simulink model "gamma_controlled_ABS"  (Simulink 7.1)
settings: Solver=ode45  SolverMode=SingleTasking  StartTime=0.0  StopTime=5  RelTol=1e-3  AbsTol=1e-6
values from neighbouring files (symbols this model uses):
  Cs = 1050.0    (= 1050)    [rho_driven_suspension.m]
  Ks = 19960.0    (= 19960)    [rho_driven_suspension.m]
  Kw = 175500.0    (= 175500)    [rho_driven_suspension.m]
  ms = 427.0    (= 427)    [rho_driven_suspension.m]
  mw = 40.0    (= 40)    [rho_driven_suspension.m]
undefined symbols (not defined in the file or in its folder): Ct
settings Model: Creator=theShunainai  LastModifiedBy=theShunainai
settings DataIOCC: LimitDataPoints=off
settings OptimizationCC: BlockReduction=off  BooleanDataType=off
settings DebuggingCC: SaveWithParameterizedLinksMsg=none  SignalResolutionControl=TryResolveAllWithWarning  SolverPrmCheckMsg=none  MultiTaskDSMMsg=warning  MultiTaskCondExecSysMsg=none  StrictBusMsg=None
settings HardwareCC: TargetUnknown=on
settings RTWCC: IncludeERTFirstTime=on

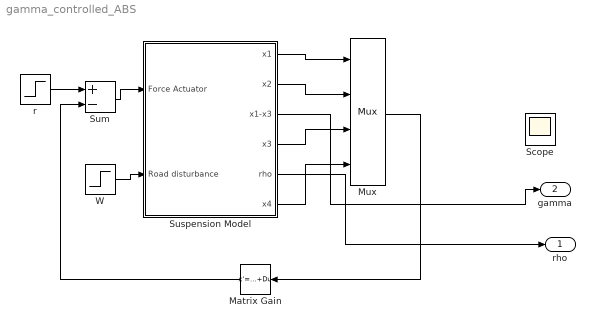
== system gamma_controlled_ABS ==
  Matrix Gain : StateSpace  Orientation=left  A=[]  B=[]  C=[]  D=K  mask(Matrix Gain){@1=-Kgamma}
      mask prompts: @1 "Gain matrix:"
      mask help: Matrix Gain.
      mask init:
      | K=@1;
      mask Help: Multiplies input vector by entered matrix to produce output vector (y=Au).
      mask Display: disp('K')
  Mux : Mux
  Scope : Scope
  Sum : Sum  Inputs=+-  SaturateOnIntegerOverflow=on  InputSameDT=on  OutDataTypeStr=Inherit: Same as first input
  Suspension Model : Subsystem
  W : Step  Time=0  After=-.1
  r : Step  Time=0  After=0
  rho : Outport  OutDataType=sfix(16)  OutScaling=2^0
  gamma : Outport  Port=2  OutDataType=sfix(16)  OutScaling=2^0
  wires:
  W/1 -> Suspension Model/2(Road disturbance)
  Sum/1 -> Suspension Model/1(Force Actuator)
  r/1 -> Sum/1
  Matrix Gain/1 -> Sum/2
  Mux/1 -> Matrix Gain/1
  Suspension Model/1(x1) -> Mux/1
  Suspension Model/2(x2) -> Mux/2
  Suspension Model/4(x3) -> Mux/3
  Suspension Model/6(x4) -> Mux/4
  Suspension Model/3(x1-x3) -> gamma/1
  Suspension Model/5(rho) -> rho/1

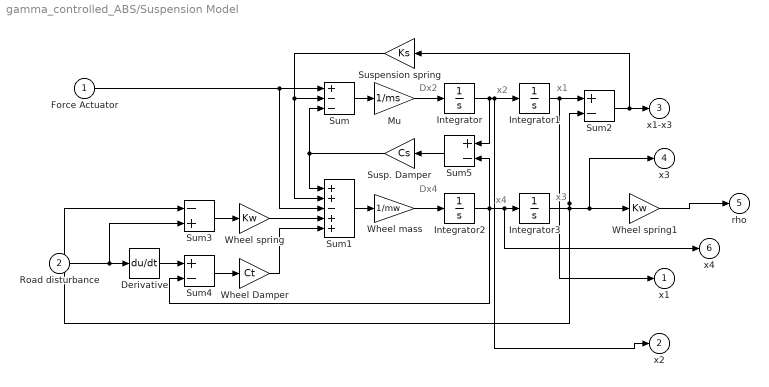
== system gamma_controlled_ABS/Suspension Model ==
  note: x3
  note: x4
  note: Dx4
  note: x1
  note: x2
  note: Dx2
  Force Actuator : Inport
  Road disturbance : Inport  Port=2
  Derivative : Derivative
  Integrator{,1..3} (4 alike) : Integrator
  Mu : Gain  Gain=1/ms  SaturateOnIntegerOverflow=on  OutDataTypeStr=Inherit: Same as input  ParamDataTypeStr=Inherit: Same as input
  Sum : Sum  Inputs=+--  SaturateOnIntegerOverflow=on  InputSameDT=on  OutDataTypeStr=Inherit: Same as first input
  Sum1 : Sum  Inputs=++-++  SaturateOnIntegerOverflow=on  InputSameDT=on  OutDataTypeStr=Inherit: Same as first input
  Sum2 : Sum  Inputs=+-  SaturateOnIntegerOverflow=on  InputSameDT=on  OutDataTypeStr=Inherit: Same as first input
  Sum3 : Sum  Inputs=-+  SaturateOnIntegerOverflow=on  InputSameDT=on  OutDataTypeStr=Inherit: Same as first input
  Sum4 : Sum  Inputs=+-  SaturateOnIntegerOverflow=on  InputSameDT=on  OutDataTypeStr=Inherit: Same as first input
  Sum5 : Sum  Orientation=left  Inputs=+-  SaturateOnIntegerOverflow=on  InputSameDT=on  OutDataTypeStr=Inherit: Same as first input
  Susp. Damper : Gain  Orientation=left  Gain=Cs  SaturateOnIntegerOverflow=on  OutDataTypeStr=Inherit: Same as input  ParamDataTypeStr=Inherit: Same as input
  Suspension spring : Gain  Orientation=left  Gain=Ks  SaturateOnIntegerOverflow=on  OutDataTypeStr=Inherit: Same as input  ParamDataTypeStr=Inherit: Same as input
  Wheel Damper : Gain  Gain=Ct  SaturateOnIntegerOverflow=on  OutDataTypeStr=Inherit: Same as input  ParamDataTypeStr=Inherit: Same as input
  Wheel mass : Gain  Gain=1/mw  SaturateOnIntegerOverflow=on  OutDataTypeStr=Inherit: Same as input  ParamDataTypeStr=Inherit: Same as input
  Wheel spring : Gain  Gain=Kw  SaturateOnIntegerOverflow=on  OutDataTypeStr=Inherit: Same as input  ParamDataTypeStr=Inherit: Same as input
  Wheel spring1 : Gain  Gain=Kw  SaturateOnIntegerOverflow=on  OutDataTypeStr=Inherit: Same as input  ParamDataTypeStr=Inherit: Same as input
  x1 : Outport  InitialOutput=0
  x2 : Outport  Port=2  InitialOutput=0
  x1-x3 : Outport  Port=3  InitialOutput=0
  x3 : Outport  Port=4  InitialOutput=0
  rho : Outport  Port=5  InitialOutput=0
  x4 : Outport  Port=6  InitialOutput=0
  wires:
  Integrator3/1 -> Sum3/1, Sum2/2, Wheel spring1/1, x3/1
  Integrator1/1 -> Sum2/1, x1/1
  Sum5/1 -> Susp. Damper/1
  Road disturbance/1 -> Derivative/1, Sum3/2
  Derivative/1 -> Sum4/1
  Force Actuator/1 -> Sum1/3, Sum/1
  Sum4/1 -> Wheel Damper/1
  Sum3/1 -> Wheel spring/1
  Wheel spring/1 -> Sum1/4
  Wheel Damper/1 -> Sum1/5
  Suspension spring/1 -> Sum1/2, Sum/2
  Sum2/1 -> x1-x3/1, Suspension spring/1
  Integrator/1 -> x2/1, Integrator1/1, Sum5/1
  Sum/1 -> Mu/1
  Mu/1 -> Integrator/1
  Susp. Damper/1 -> Sum/3, Sum1/1
  Integrator2/1 -> Sum5/2, Sum4/2, Integrator3/1, x4/1
  Sum1/1 -> Wheel mass/1
  Wheel mass/1 -> Integrator2/1
  Wheel spring1/1 -> rho/1
